simulink model "WEEK2QUESTION1"  (R2020a)
settings: Solver=VariableStepAuto  StartTime=0.0  StopTime=10.0  RelTol=1e-3
settings Model: Creator=anjal  LastModifiedBy=anjal

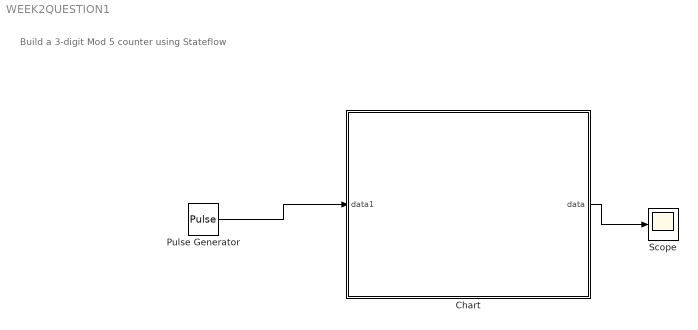
== system WEEK2QUESTION1 ==
  note: Build a 3-digit Mod 5 counter using Stateflow
  Chart : Stateflow chart  TreatAsAtomicUnit=on
  Pulse Generator : DiscretePulseGenerator  PulseType=Time based  Period=10  PulseWidth=5
  Scope : Scope
  wires:
  Pulse Generator/1 -> Chart/1(data1)
  Chart/1(data) -> Scope/1

== stateflow chart WEEK2QUESTION1/Chart ==
  state Counter
    state FirstDigit
      state Zero
        en:d1=0;
      state One
        en:d1=1;
        en:clear=0;
      Counter.FirstDigit.Zero -> Counter.FirstDigit.One
      (default) -> Counter.FirstDigit.Zero
      Counter.FirstDigit.One -> Counter.FirstDigit.Zero
    state SecondDigit
      state Zero
        en:d2=0;
      state One2
        en:d3=1;
        en:clear=1;
      Counter.SecondDigit.Zero -> One2
      (default) -> Counter.SecondDigit.Zero
      One2 -> Counter.SecondDigit.Zero
    state ThirdDigit
      state Zero
        en:d3=0;
      state One
        en:d3=1;
        en:clear=1;
      Counter.ThirdDigit.Zero -> Counter.ThirdDigit.One
      (default) -> Counter.ThirdDigit.Zero
      Counter.ThirdDigit.One -> Counter.ThirdDigit.Zero
    (default) -> FirstDigit [order 1]
    (default) -> SecondDigit [order 3]
    (default) -> ThirdDigit [order 2]
  (default) -> Counter
  data: data output; data1 input
